simulink model "Problem_2_2slx"  (R2013a)
settings: Solver=ode45  StartTime=0.0  StopTime=20  RelTol=1e-3
undefined symbols (not defined in the file): A, J, Ka, Kb, Km, R
settings Model: Creator=Samanth  LastModifiedBy=Samanth
settings DebuggingCC: AlgebraicLoopMsg=none  SolverPrmCheckMsg=none

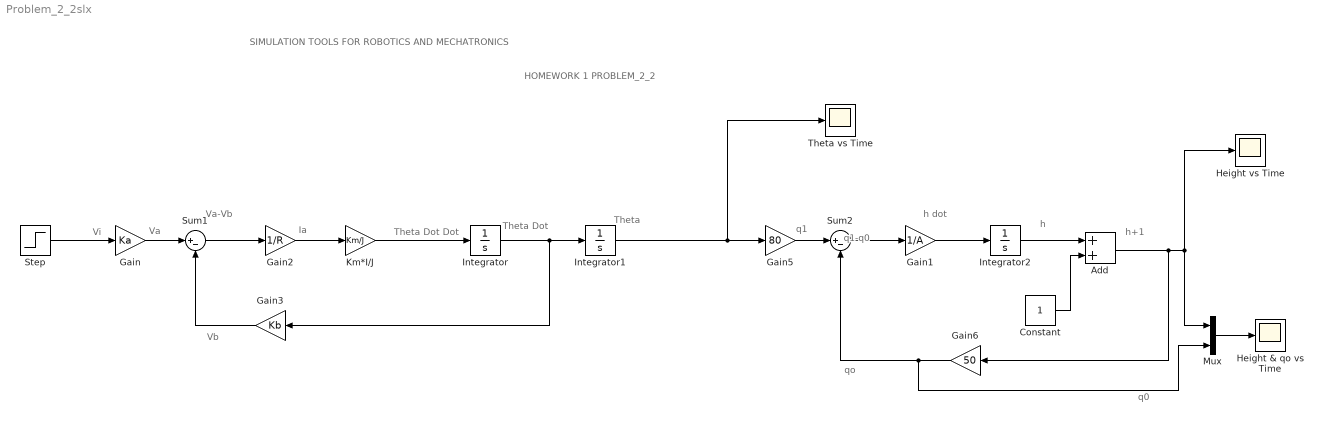
== system Problem_2_2slx ==
  note: SIMULATION TOOLS FOR ROBOTICS AND MECHATRONICS
  note: q0
  note: h+1
  note: q1-q0
  note: qo
  note: q1
  note: Ia
  note: Va-Vb
  note: Vb
  note: Va
  note: h
  note: h dot
  note: Theta
  note: Theta Dot
  note: Theta Dot Dot
  note: HOMEWORK 1
      | PROBLEM_2_2
  note: Vi
  Add : Sum
  Constant : Constant
  Gain : Gain  Gain=Ka
  Gain1 : Gain  Gain=1/A
  Gain2 : Gain  Gain=1/R
  Gain3 : Gain  Gain=Kb
  Gain5 : Gain  Gain=80
  Gain6 : Gain  Gain=50
  Height & qo vs Time : Scope
  Height vs Time : Scope
  Integrator : Integrator
  Integrator1 : Integrator
  Integrator2 : Integrator
  Km*I/J : Gain  Gain=Km/J
  Mux : Mux  Inputs=2
  Step : Step  Time=0  After=1.5  SampleTime=0
  Sum1 : Sum  Inputs=|+-
  Sum2 : Sum  Inputs=|+-
  Theta vs Time : Scope
      settings: SaveName=ScopeData2
  wires:
  Gain/1 -> Sum1/1
  Sum1/1 -> Gain2/1
  Gain2/1 -> Km*I/J/1
  Gain3/1 -> Sum1/2
  Km*I/J/1 -> Integrator/1
  Integrator/1 -> Gain3/1, Integrator1/1
  Gain6/1 -> Mux/2, Sum2/2
  Step/1 -> Gain/1
  Gain5/1 -> Sum2/1
  Sum2/1 -> Gain1/1
  Gain1/1 -> Integrator2/1
  Integrator1/1 -> Theta vs Time/1, Gain5/1
  Integrator2/1 -> Add/1
  Add/1 -> Gain6/1, Mux/1, Height vs Time/1
  Constant/1 -> Add/2
  Mux/1 -> Height & qo vs Time/1
